simulink model "CASB185Project"  (R2020b)
settings: Solver=VariableStepAuto  StartTime=0.0  StopTime=1050  RelTol=1e-3
settings Model: Creator=rubsy  LastModifiedBy=rubsy

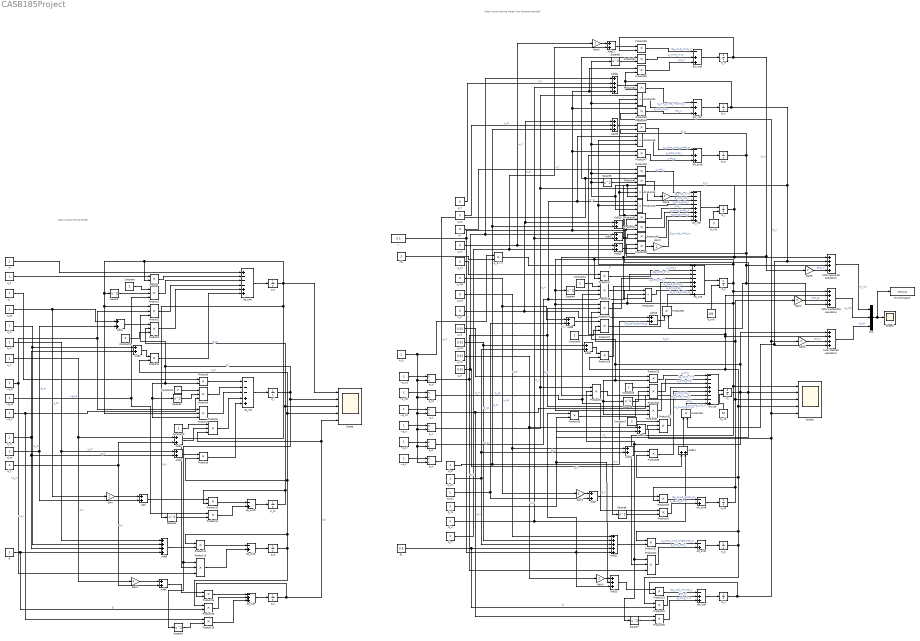
== system CASB185Project ==
  note: Mass-Action Pairing Model
  note: Mass-Action Pairing Model (non-dimensionalized)
  A_0 : Constant
  A_0 * Π : Product
  Add{,1..4,6..11,14..18,21} (17 alike) : Sum
  Add12 : Sum  Inputs=+++++
  Add13 : Sum  Inputs=+++
  Add19 : Sum  Inputs=+++
  Add20 : Sum  Inputs=++++
  Add5 : Sum  Inputs=++++
  Constant{,1..7} (8 alike) : Constant  Value=2
  Gain{,1..9} (10 alike) : Gain  Gain=2
  Mux : Mux  Inputs=3
  N_i : Integrator  InitialConditionSource=external
  N_i(0) : Constant  Value=10
  N_ii : Integrator
  N_ir : Integrator
  N_r : Integrator  InitialConditionSource=external
  N_r(0) : Constant  Value=0
  N_rr : Integrator
  N_s : Integrator  InitialConditionSource=external
  N_s(0) : Constant  Value=100
  N_si : Integrator
  N_sr : Integrator
  N_ss : Integrator
  Product{,4..5,9..12,14..17,19..21,23..25,28..29,33,35..36,38..42,45..47,49..50,52..55} (36 alike) : Product
  Product{1..3,6..8,13,18,22,26..27,30..32,34,37,43..44,48,51} (20 alike) : Product  Inputs=3
  Scope : Scope  NumInputPorts=5
  Scope1 : Scope  NumInputPorts=5
  Scope2 : Scope
  Square{,1..9} (10 alike) : Math  Operator=square  SaturateOnIntegerOverflow=on
  To Workspace : ToWorkspace  VariableName=simout  SaveFormat=Structure With Time  SampleTime=-1
  a_ii : Product  Inputs=*/
  a_ir : Product  Inputs=*/
  a_rr : Product  Inputs=*/
  a_si : Product  Inputs=*/
  a_sr : Product  Inputs=*/
  a_ss : Product  Inputs=*/
  dN_i/dt : Sum  Inputs=---++--+
  dN_ii/dt : Sum  Inputs=-++
  dN_ir/dt : Sum  Inputs=-++
  dN_r/dt : Sum  Inputs=----++++
  dN_rr/dt : Sum  Inputs=-++
  dN_s/dt : Sum  Inputs=+---++-+
  dN_si/dt : Sum  Inputs=-+
  dN_sr/dt : Sum  Inputs=-++
  dN_ss/dt : Sum  Inputs=-+
  d_ii : Constant
  d_ii1 : Constant
  d_ir : Constant
  d_rr : Constant
  d_si : Constant
  d_si1 : Constant
  d_sr : Constant
  d_ss : Constant
  d_ss1 : Constant
  dρ_i/dt : Sum  Inputs=---++
  dρ_ii/dt : Sum  Inputs=-++
  dρ_s/dt : Sum  Inputs=+---++
  dρ_si/dt : Sum  Inputs=-+
  dρ_ss/dt : Sum  Inputs=-+
  total infected population : Sum  Inputs=++++
  total recovered population : Sum  Inputs=++++
  total susceptible population : Sum  Inputs=++++
  y : Constant  Value=0.1
  ~a_ii : Constant
  ~a_ii1 : Constant
  ~a_ir : Constant
  ~a_rr : Constant
  ~a_si : Constant
  ~a_si1 : Constant
  ~a_sr : Constant
  ~a_ss : Constant
  ~a_ss1 : Constant
  Π : Constant
  Π1 : Constant  Value=2
  β : Constant
  β1 : Constant  Value=0.5
  μ_i : Constant
  μ_i1 : Constant  Value=0.01
  μ_ii : Constant
  μ_ii1 : Constant  Value=0.01
  μ_ir : Constant  Value=0.01
  μ_is : Constant
  μ_is1 : Constant  Value=0.01
  μ_r : Constant  Value=0
  μ_ri : Constant  Value=0
  μ_rr : Constant  Value=0
  μ_rs : Constant  Value=0
  μ_s : Constant
  μ_s1 : Constant  Value=0
  μ_si : Constant
  μ_si1 : Constant  Value=0
  μ_sr : Constant  Value=0
  μ_ss : Constant
  μ_ss1 : Constant  Value=0
  ρ_i : Integrator
  ρ_ii : Integrator
  ρ_s : Integrator
  ρ_si : Integrator
  ρ_ss : Integrator
  wires:
  Π/1 -> dρ_s/dt/1
  Product/1 -> dρ_s/dt/2
  μ_s/1 -> Product/1
  ρ_s/1 -> Product13/2, Square2/1, Product/2, Product7/2, Product2/1, Square/1, Scope/1  "ρ_s"
  Product1/1 -> dρ_s/dt/3
  Constant/1 -> Product1/1
  Square/1 -> Product1/2
  ~a_ss/1 -> Product11/1, Product1/3  "~a_ss"
  ~a_si/1 -> Product13/3, Product7/1, Product2/2  "~a_si"
  ρ_i/1 -> Product2/3, Product7/3, Square1/1, Product5/2, Product13/1, Square3/1, Scope/2  "ρ_i"
  Product2/1 -> dρ_s/dt/4
  μ_ss/1 -> Gain/1, Add1/1  "μ_ss"
  d_ss/1 -> Add1/2, Add/2  "d_ss"
  Add1/1 -> Product3/1
  Constant1/1 -> Product3/3
  Product3/1 -> dρ_s/dt/5
  μ_is/1 -> Add2/1, Add5/2  "μ_is"
  d_si/1 -> Add5/3, Add4/2, Add2/2  "d_si"
  Add2/1 -> Product4/1
  Product4/1 -> dρ_s/dt/6
  dρ_s/dt/1 -> ρ_s/1
  Product5/1 -> dρ_i/dt/1
  μ_i/1 -> Product5/1
  Product6/1 -> dρ_i/dt/2
  Constant2/1 -> Product6/1
  ~a_ii/1 -> Product16/1, Product6/3  "~a_ii"
  Square1/1 -> Product6/2
  Product7/1 -> dρ_i/dt/3
  dρ_i/dt/1 -> ρ_i/1
  Product8/1 -> dρ_i/dt/4
  Constant3/1 -> Product8/1
  Add3/1 -> Product8/2
  dρ_ss/dt/1 -> ρ_ss/1
  ρ_ss/1 -> Product10/2, Product3/2, Scope/3  "ρ_ss"
  dρ_si/dt/1 -> ρ_si/1
  ρ_si/1 -> Product15/1, Product12/1, Product9/2, Product4/2, Scope/4  "ρ_si"
  dρ_ii/dt/1 -> ρ_ii/1
  ρ_ii/1 -> Product14/2, Product8/3, Scope/5  "ρ_ii"
  μ_ii/1 -> Gain1/1, Add3/1  "μ_ii"
  d_ii/1 -> Add6/2, Add3/2  "d_ii"
  Product9/1 -> dρ_i/dt/5
  Add4/1 -> Product9/1
  μ_si/1 -> Add5/1, Add4/1  "μ_si"
  Product10/1 -> dρ_ss/dt/1
  Add/1 -> Product10/1
  Gain/1 -> Add/1
  Product11/1 -> dρ_ss/dt/2
  Square2/1 -> Product11/2
  Product12/1 -> dρ_si/dt/1
  Add5/1 -> Product12/2
  β/1 -> Product15/2, Add5/4  "β"
  Product13/1 -> dρ_si/dt/2
  Product14/1 -> dρ_ii/dt/1
  Gain1/1 -> Add6/1
  Add6/1 -> Product14/1
  Product15/1 -> dρ_ii/dt/2
  Product16/1 -> dρ_ii/dt/3
  Square3/1 -> Product16/2
  Square7/1 -> Product25/2
  Product23/1 -> dN_ii/dt/1  "(2μ_ii+d_ii+y)*N_ii"
  Square6/1 -> Product20/2
  β1/1 -> Product24/2, Add12/4  "β"
  Product19/1 -> dN_ss/dt/1  "(2μ_ss+d_ss)*N_ss"
  Product24/1 -> dN_ii/dt/2  "β*N_si"
  dN_ii/dt/1 -> N_ii/1
  Add13/1 -> Product23/1
  μ_si1/1 -> Add12/1, Add11/1  "μ_si"
  N_ii/1 -> Product23/2, Product32/3, Gain5/1, Product50/2, Scope1/5  "N_ii"
  Product25/1 -> dN_ii/dt/3  "a_ii*(N_i)^2"
  Add12/1 -> Product21/2
  dN_si/dt/1 -> N_si/1
  Add7/1 -> Product19/1
  Product30/1 -> dN_i/dt/2  "2a_ii*(N_i)^2"
  Product32/1 -> dN_i/dt/4  "2(μ_ii+d_ii)*N_ii"
  N_ss/1 -> Product19/2, Product27/2, Gain4/1, Scope1/3  "N_ss"
  Add10/1 -> Product32/2
  Add8/1 -> Product27/1
  d_si1/1 -> Add9/2, Add11/2, Add12/3  "d_si"
  Product33/1 -> dN_i/dt/5  "(μ_si+d_si)*N_si"
  d_ss1/1 -> Add8/2, Add7/2  "d_ss"
  N_si/1 -> Product24/1, Product21/1, Product33/2, Product28/2, total susceptible population/2, Product47/2, total infected population/2, Scope1/4  "N_si"
  dN_i/dt/1 -> N_i/1
  μ_ss1/1 -> Gain2/1, Add8/1  "μ_ss"
  a_ss/1 -> Product18/3, Product20/1  "a_ss"
  Constant5/1 -> Product27/3
  Product26/1 -> dN_s/dt/4  "a_si*N_s*N_i"
  Product27/1 -> dN_s/dt/5  "2(μ_ss+d_ss)*N_ss"
  Product29/1 -> dN_i/dt/1  "μ_i*N_i"
  μ_s1/1 -> Product17/1
  Product28/1 -> dN_s/dt/6  "(μ_is+d_si)*N_si"
  Gain2/1 -> Add7/1
  Product18/1 -> dN_s/dt/3  "2a_ss*N_s^2"
  Constant7/1 -> Product32/1
  Square4/1 -> Product18/2
  dN_ss/dt/1 -> N_ss/1
  Add11/1 -> Product33/1
  Constant4/1 -> Product18/1
  N_i/1 -> Product34/2, Product22/1, Square7/1, Product44/2, Product51/2, Product42/1, Product35/2, Scope1/2, total infected population/1, Product26/3, Product31/3, Square5/1, Product29/2  "N_i"
  Product21/1 -> dN_si/dt/1  "(μ_is+μ_si+d_si+β+y)*N_si"
  a_ii/1 -> Product30/3, Product25/1  "a_ii"
  μ_is1/1 -> Add9/1, Add12/2  "μ_is"
  Product31/1 -> dN_i/dt/3  "a_si*N_s*N_i"
  a_si/1 -> Product31/1, Product26/2, Product22/3  "a_si"
  N_s/1 -> Scope1/1, Product22/2, Product37/2, Square6/1, total susceptible population/1, Product48/2, Product43/2, Product17/2, Product31/2, Product26/1, Square4/1  "N_s"
  Product20/1 -> dN_ss/dt/2  "a_ss*(N_s)^2"
  d_ii1/1 -> Add13/2, Add10/2  "d_ii"
  Product22/1 -> dN_si/dt/2  "a_si*N_s*N_i"
  Gain3/1 -> Add13/1
  Constant6/1 -> Product30/1
  Add9/1 -> Product28/1
  dN_s/dt/1 -> N_s/1
  A_0 * Π/1 -> dN_s/dt/1  "Π"
  μ_ii1/1 -> Gain3/1, Add10/1  "μ_ii"
  μ_i1/1 -> Product29/1
  Square5/1 -> Product30/2
  Product17/1 -> dN_s/dt/2  "μ_s*N_s"
  Π1/1 -> A_0 * Π/2
  A_0/1 -> A_0 * Π/1, a_si/2, a_ss/2, a_rr/2, a_sr/2, a_ir/2, a_ii/2
  ~a_si1/1 -> a_si/1
  ~a_ss1/1 -> a_ss/1
  ~a_ii1/1 -> a_ii/1
  N_s(0)/1 -> N_s/2
  N_i(0)/1 -> N_i/2
  total susceptible population/1 -> Mux/2  "N_s(t)"
  Gain4/1 -> total susceptible population/3  "2*N_ss"
  total infected population/1 -> Mux/3  "N_i(t)"
  Gain5/1 -> total infected population/3  "2*N_ii"
  Mux/1 -> To Workspace/1, Scope2/1
  dN_r/dt/1 -> N_r/1
  N_r(0)/1 -> N_r/2
  total recovered population/1 -> Mux/1  "N_r(t)"
  N_r/1 -> total recovered population/1, Product37/3, Product34/3, Product44/3, Square9/1, Product51/3, Product48/3, Product46/2, Square8/1, Product43/3  "N_r"
  N_ir/1 -> Product53/2, Product52/2, Product36/2, total infected population/4, total recovered population/2, Product40/2  "N_ir"
  N_sr/1 -> Product49/2, Product41/2, Product38/2, total susceptible population/4, total recovered population/3  "N_sr"
  Gain6/1 -> total recovered population/4  "2*N_rr"
  dN_sr/dt/1 -> N_sr/1
  N_rr/1 -> Product55/2, Product39/1, Gain6/1  "N_rr"
  Product46/1 -> dN_r/dt/1  "μ_r*N_r"
  Gain8/1 -> dN_r/dt/2  "2a_rr(N_r)^2"
  Product37/1 -> dN_s/dt/7  "a_sr*N_s*N_r"
  Product38/1 -> dN_s/dt/8  "(μ_sr+d_sr)*N_sr"
  Product44/1 -> dN_r/dt/3  "a_ir*N_i*N_r"
  Product43/1 -> dN_r/dt/4  "a_sr*N_s*N_r"
  Product42/1 -> dN_r/dt/5  "y*N_i"
  Product41/1 -> dN_r/dt/6  "(μ_sr+d_sr)*N_sr"
  Product40/1 -> dN_r/dt/7  "(μ_ir+d_ir)*N_ir"
  Gain7/1 -> dN_r/dt/8  "2(μ_rr+d_rr)*N_rr"
  Product49/1 -> dN_sr/dt/1  "(μ_sr+μ_rs+d_sr)*N_sr"
  Product48/1 -> dN_sr/dt/2  "a_sr*N_s*N_r"
  Product47/1 -> dN_sr/dt/3  "y*N_si"
  dN_ir/dt/1 -> N_ir/1
  Product52/1 -> dN_ir/dt/1  "(μ_ir+μ_ri+d_ir+y)*N_ir"
  Product50/1 -> dN_ir/dt/3  "y*N_ii"
  Product51/1 -> dN_ir/dt/2  "a_ir*N_i*N_r"
  dN_rr/dt/1 -> N_rr/1
  Product55/1 -> dN_rr/dt/1  "(2μ_rr+d_rr)*N_rr"
  Product54/1 -> dN_rr/dt/2  "a_rr*(N_r)^2"
  Product53/1 -> dN_rr/dt/3  "y*N_ir"
  Product34/1 -> dN_i/dt/6  "a_ir*N_i*N_r"
  Product35/1 -> dN_i/dt/7  "y*N_i"
  Product36/1 -> dN_i/dt/8  "(μ_ir+d_ir)N_ir"
  y/1 -> Product53/1, Add20/4, Product50/1, Product47/1, Product42/2, Product35/1, Add13/3, Add12/5  "y"
  ~a_ir/1 -> a_ir/1
  a_ir/1 -> Product34/1, Product51/1, Product44/1  "a_ir"
  Add14/1 -> Product36/1
  μ_ir/1 -> Add20/1, Add17/1, Add14/1  "μ_ir"
  d_ir/1 -> Add14/2, Add20/3, Add17/2  "d_ir"
  ~a_sr/1 -> a_sr/1
  a_sr/1 -> Product48/1, Product43/1, Product37/1  "a_sr"
  Add16/1 -> Product38/1
  μ_sr/1 -> Add19/1, Add18/1, Add16/1  "μ_sr"
  d_sr/1 -> Add19/3, Add18/2, Add16/2  "d_sr"
  Product39/1 -> Gain7/1
  Add15/1 -> Product39/2
  μ_rr/1 -> Gain9/1, Add15/1  "μ_rr"
  d_rr/1 -> Add21/2, Add15/2  "d_rr"
  Add17/1 -> Product40/1
  Add18/1 -> Product41/1
  Square8/1 -> Product45/2
  Product45/1 -> Gain8/1
  ~a_rr/1 -> a_rr/1
  a_rr/1 -> Product54/1, Product45/1  "a_rr"
  μ_r/1 -> Product46/1  "μ_r"
  Add19/1 -> Product49/1
  μ_rs/1 -> Add19/2  "μ_rs"
  Add20/1 -> Product52/1
  μ_ri/1 -> Add20/2  "μ_ri"
  Square9/1 -> Product54/2
  Add21/1 -> Product55/1
  Gain9/1 -> Add21/1
